simulink model "Controller5"  (R2021b)
settings: Solver=VariableStepAuto  StartTime=0.0  StopTime=10.0  RelTol=1e-3
libraries: simulink_extras x1
settings Model: Creator=david  LastModifiedBy=david

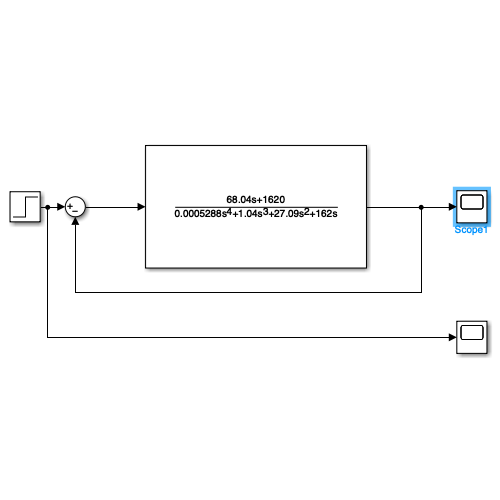
[thumbnail: Simulink's stored preview of the top-level diagram]
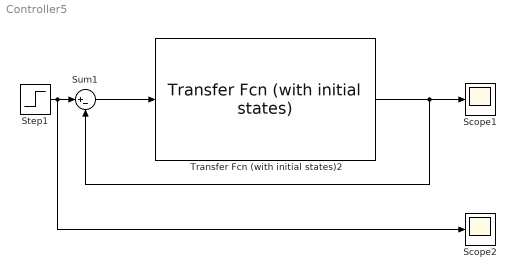
== system Controller5 ==
  Scope1 : Scope
  Scope2 : Scope
  Step1 : Step  SampleTime=0
  Sum1 : Sum  Inputs=|+-
  Transfer Fcn (with initial states)2 : simulink_extras/Additional Linear/Transfer Fcn (with initial states)  N=[68.04 1620]  D=[.0005288 1.04 27.09 162 0]  X0=0
  wires:
  Sum1/1 -> Transfer Fcn (with initial states)2/1
  Transfer Fcn (with initial states)2/1 -> Scope1/1, Sum1/2
  Step1/1 -> Scope2/1, Sum1/1
